simulink model "posLQR"  (R2023a)
settings: Solver=ode4  StartTime=0.0  StopTime=inf  FixedStep=0.002  RelTol=1e-3  EnableMultiTasking=on
PostLoadFcn:
  | qc_set_target_type(getConfigSet(bdroot, 'QUARC Default Target Configuration'));
values from neighbouring files (symbols this model uses):
  A = M^-1*Ahat    [Init.m]
  B = M^-1*Bhat    [Init.m]
  C = eye(4)    [Init.m]
  D = zeros(4,1)    [Init.m]
  wc = 150    [Init.m]
undefined symbols (not defined in the file or in its folder): HIL, Kc
libraries: quarc_library x5, simulink_extras x1
settings Model: SimulationMode=external  ExtModeTrigDuration=10000  Creator=MLevis  LastModifiedBy=quarc_user
settings SolverCC: AlgebraicLoopSolver=TrustRegion  PositivePriorityOrder=on  AutoInsertRateTranBlk=on
settings DataIOCC: LimitDataPoints=on  SaveFormat=Array  SignalLoggingSaveFormat=ModelDataLogs  ReturnWorkspaceOutputs=off
settings OptimizationCC: ExpressionDepthLimit=2147483647  InitFltsAndDblsToZero=on
settings DebuggingCC: SaveWithParameterizedLinksMsg=none  UnderspecifiedInitializationDetection=Classic  MergeDetectMultiDrivingBlocksExec=none  SolverPrmCheckMsg=warning  MultiTaskDSMMsg=warning  MultiTaskCondExecSysMsg=none  FcnCallInpInsideContextMsg=warning  UnconnectedInputMsg=warning  UnconnectedOutputMsg=warning  UnconnectedLineMsg=warning  StateNameClashWarn=warning  SFUnexpectedBacktrackingDiag=warning  SFNoUnconditionalDefaultTransitionDiag=warning  SFExecutionAtInitializationDiag=none  ArithmeticOperatorsInVariantConditions=warning
settings ModelReferenceCC: EnableRefExpFcnMdlSchedulingChecks=on  PropagateSignalLabelsOutOfModel=off
settings SFSimCC: SimUseLocalCustomCode=off  CustomCodeUndefinedFunction=UseInterfaceOnly
settings RTWCC: Description=QUARC Win64 Target Using Toolchain  SystemTargetFile=quarc_win64.tlc  TemplateMakefile=quarc_default_tmf  RTWUseLocalCustomCode=off  Toolchain=QUARC win64 | nmake (64-bit Windows)  BuildConfiguration=Faster Runs  DLArmComputeVersion=19.05
settings CodeAppCC: StateflowObjectComments=on
settings STFCustomTargetCC: TargetLangStandard=C89/C90 (ANSI)  SystemTargetFile=quarc_win64.tlc
settings GRTTargetCC: TargetLangStandard=C89/C90 (ANSI)  ParMdlRefBuildCompliant=off  CompOptLevelCompliant=off  CombineOutputUpdateFcns=off  MatFileLogging=off  CPPClassGenCompliant=off  GRTInterface=on  ExtMode=on  ExtModeMexFile=quarc_comm
settings ConfigComp: CovMetricSettings=dw  CovSaveCumulativeToWorkspaceVar=on  CovSaveSingleToWorkspaceVar=on  CovExternalEMLEnable=off

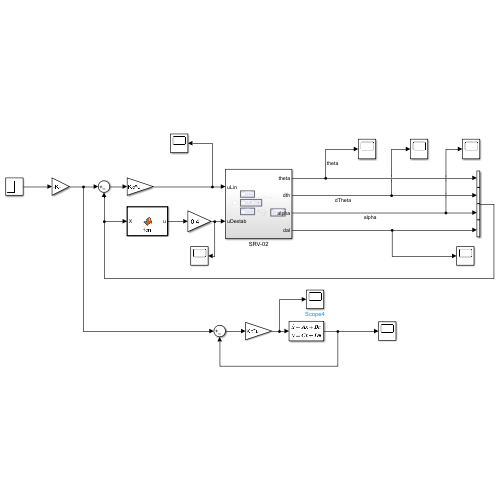
[thumbnail: Simulink's stored preview of the top-level diagram]
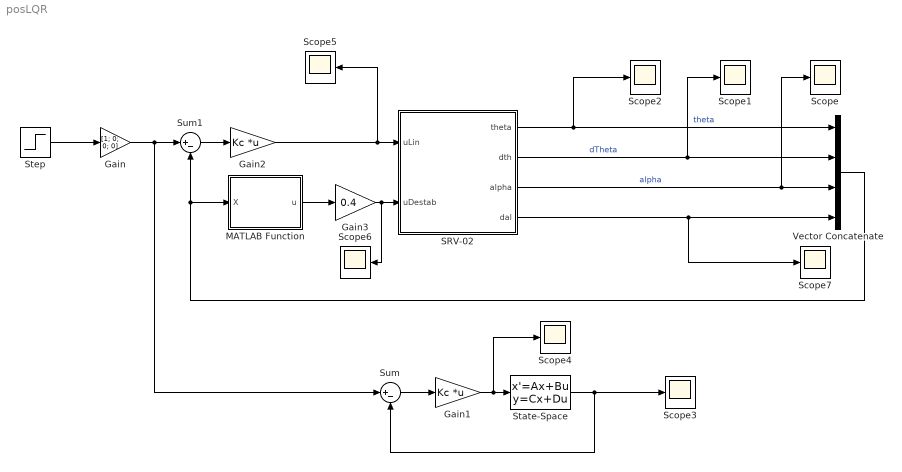
== system posLQR ==
  Gain : Gain  Gain=[1; 0; 0; 0]
  Gain1 : Gain  Gain=Kc  Multiplication=Matrix(K*u)
  Gain2 : Gain  Gain=Kc  Multiplication=Matrix(K*u)
  Gain3 : Gain  Gain=0.4
  MATLAB Function : MATLAB Function  TreatAsAtomicUnit=on
  SRV-02 : Subsystem
  Scope{,1..7} (8 alike) : Scope
  State-Space : StateSpace  A=A  B=B  C=C  D=D  InitialCondition=0
  Step : Step  After=0  SampleTime=0
  Sum : Sum  Inputs=|+-
  Sum1 : Sum  Inputs=|+-
  Vector Concatenate : Concatenate  NumInputs=4
  wires:
  SRV-02/3(alpha) -> Scope/1, Vector Concatenate/3  "alpha"
  SRV-02/2(dth) -> Scope1/1, Vector Concatenate/2  "dTheta"
  Step/1 -> Gain/1
  SRV-02/1(theta) -> Vector Concatenate/1, Scope2/1  "theta"
  Gain/1 -> Sum/1, Sum1/1
  Sum/1 -> Gain1/1
  Gain1/1 -> Scope4/1, State-Space/1
  State-Space/1 -> Sum/2, Scope3/1
  Sum1/1 -> Gain2/1
  Gain2/1 -> Scope5/1, SRV-02/1(uLin)
  Vector Concatenate/1 -> Sum1/2, MATLAB Function/1(X)
  MATLAB Function/1(u) -> Gain3/1
  Gain3/1 -> Scope6/1, SRV-02/2(uDestab)
  SRV-02/4(dal) -> Scope7/1, Vector Concatenate/4

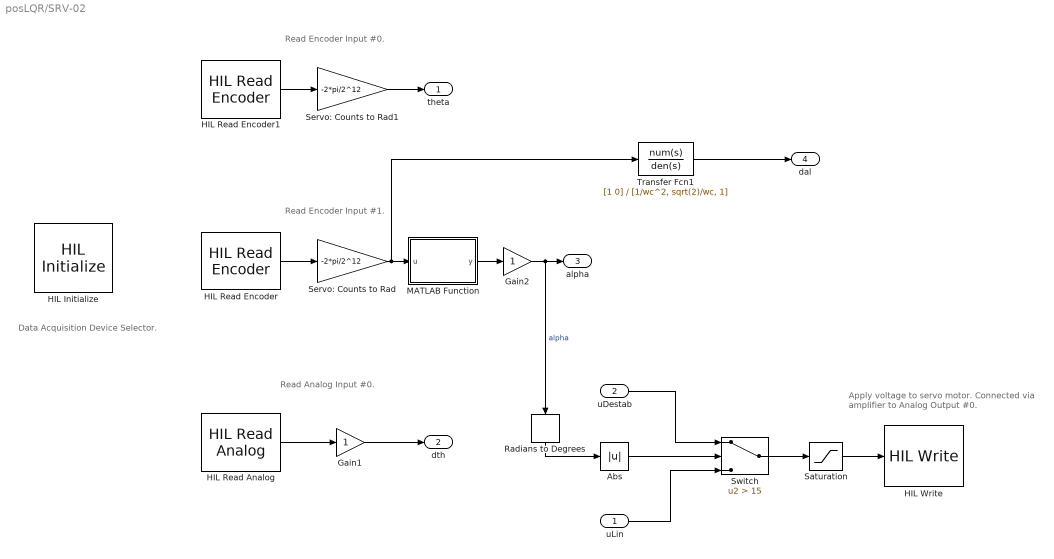
== system posLQR/SRV-02 ==
  note: Apply voltage to servo motor.
      | Connected via amplifier to Analog Output #0.
  note: Read Analog Input #0.
  note: Read Encoder Input #1.
  note: Data Acquisition Device Selector.
  note: Read Encoder Input #0.
  uLin : Inport
  uDestab : Inport  Port=2
  Abs : Abs  SaturateOnIntegerOverflow=off
  Gain1 : Gain
  Gain2 : Gain
  HIL Initialize : quarc_library/Data Acquisition/Generic/Configuration/HIL Initialize  object_name=HIL-1  board_type=q2_usb  board_number=0  board_options=d0=digital;d1=digital;led=auto;update_rate=normal;decimation=1  exclusive=off  active=off  hardware_clocks=[0]  clock_modes=[]  initial_clock_frequencies=[]  set_clock_params_at_start=off  set_clock_params_at_switch_in=off  set_clock_frequencies_at_start=off  set_clock_frequencies_at_switch_in=off  analog_input_channels=[0:1]  analog_input_configurations=[]  analog_input_maximums=10  analog_input_minimums=-10  set_analog_input_params_at_start=on  set_analog_input_params_at_switch_in=off  analog_output_channels=[0:1]  analog_output_maximums=10  analog_output_minimums=-10  initial_analog_outputs=[0]  final_analog_outputs=[0]  watchdog_analog_outputs=0  set_analog_output_params_at_start=on  set_analog_output_params_at_switch_in=off  set_analog_outputs_at_start=on  set_analog_outputs_at_switch_in=off  set_analog_outputs_at_terminate=on  set_analog_outputs_at_switch_out=off  set_analog_outputs_on_watchdog=off  digital_input_channels=[]  digital_output_channels=[]  digital_output_configuration=[]  initial_digital_outputs=[1]  final_digital_outputs=[1]  watchdog_digital_outputs=[1]  set_digital_output_params_at_start=off  set_digital_output_params_at_switch_in=off  set_digital_outputs_at_start=on  set_digital_outputs_at_switch_in=off  set_digital_outputs_at_terminate=on  set_digital_outputs_at_switch_out=off  set_digital_outputs_on_watchdog=off  encoder_channels=[0:1]  quadrature=[4]  encoder_filter_frequency=[]  initial_encoder_counts=[0]  set_encoder_params_at_start=on  set_encoder_params_at_switch_in=off  set_encoder_counts_at_start=on  set_encoder_counts_at_switch_in=off  pwm_channels=[]  pwm_modes=[0]  pwm_frequency=1/0.020  pwm_configuration=[]  pwm_alignment=[]  pwm_polarity=[]  pwm_leading_deadband=[]  pwm_trailing_deadband=[]  initial_pwm_outputs=[0]  final_pwm_outputs=[0]  watchdog_pwm_outputs=[0]  set_pwm_params_at_start=on  set_pwm_params_at_switch_in=off  set_pwm_outputs_at_start=on  set_pwm_outputs_at_switch_in=off  set_pwm_outputs_at_terminate=on  set_pwm_outputs_at_switch_out=off  set_pwm_outputs_on_watchdog=off  other_output_channels=[]  initial_other_outputs=[]  final_other_outputs=[]  watchdog_other_outputs=[]  set_other_outputs_at_start=off  set_other_outputs_at_switch_in=off  set_other_outputs_at_terminate=off  set_other_outputs_at_switch_out=off  set_other_outputs_on_watchdog=off
  HIL Read Analog : quarc_library/Data Acquisition/Generic/Immediate I//O/HIL Read Analog  object_name=HIL-1  channels=[0]  sample_time=qc_get_step_size  active=on  vector_output=off
  HIL Read Encoder : quarc_library/Data Acquisition/Generic/Immediate I//O/HIL Read Encoder  object_name=HIL-1  channels=1  sample_time=qc_get_step_size  active=on  vector_output=off  data_type_mode=Inherit via back propagation  data_type=double
  HIL Read Encoder1 : quarc_library/Data Acquisition/Generic/Immediate I//O/HIL Read Encoder  object_name=HIL-1  channels=0  sample_time=qc_get_step_size  active=on  vector_output=off  data_type_mode=Inherit via back propagation  data_type=double
  HIL Write : quarc_library/Data Acquisition/Generic/Immediate I//O/HIL Write  Tag=unassigned  object_name=HIL-1  analog_channels=0  pwm_channels=[]  digital_channels=[]  other_channels=[]  sample_time=-1  active=off  vector_input=off
  MATLAB Function : MATLAB Function  TreatAsAtomicUnit=on
  Radians to Degrees : simulink_extras/Transformations/Radians to Degrees
  Saturation : Saturate  UpperLimit=10  LowerLimit=-10
  Servo: Counts to Rad : Gain  Gain=-2*pi/2^12
  Servo: Counts to Rad1 : Gain  Gain=-2*pi/2^12
  Switch : Switch  Criteria=u2 > Threshold  Threshold=15  SaturateOnIntegerOverflow=off  InputSameDT=off
  Transfer Fcn1 : TransferFcn  Numerator=[1 0]  Denominator=[1/wc^2, sqrt(2)/wc, 1]  ParameterTunability=Unconstrained
  theta : Outport
  dth : Outport  Port=2
  alpha : Outport  Port=3
  dal : Outport  Port=4
  wires:
  HIL Read Encoder/1 -> Servo: Counts to Rad/1
  HIL Read Analog/1 -> Gain1/1
  Servo: Counts to Rad/1 -> Transfer Fcn1/1, MATLAB Function/1(u)
  Saturation/1 -> HIL Write/1
  Switch/1 -> Saturation/1
  Gain1/1 -> dth/1
  Servo: Counts to Rad1/1 -> theta/1
  HIL Read Encoder1/1 -> Servo: Counts to Rad1/1
  MATLAB Function/1(y) -> Gain2/1
  Abs/1 -> Switch/2
  Gain2/1 -> alpha/1, Radians to Degrees/1  "alpha"
  Radians to Degrees/1 -> Abs/1
  uLin/1 -> Switch/3
  uDestab/1 -> Switch/1
  Transfer Fcn1/1 -> dal/1

== matlab function posLQR/SRV-02/MATLAB Function ==
  data: u input; y output
function y = modAlpha(u)

y = mod(u,2*pi) - pi;

== matlab function posLQR/MATLAB Function ==
  data: X input; u output
function u = fcn(X)

alpha = X(3);
alphaDot = X(4);

epsilon = 0.1;

if abs(alphaDot) < epsilon && abs(alpha) > pi - epsilon
    u = 5;
else
    u = cos(alpha)*alphaDot;
end
